simulink model "Wheelspeed_Logik_compatible"  (R2022b)
settings: Solver=FixedStepAuto  StartTime=0.0  StopTime=10.0  FixedStep=0.0001  RelTol=1e-3
libraries: simulink x2
settings Model: Creator=finneinhoff  LastModifiedBy=finneinhoff
settings OptimizationCC: ReuseModelBlockBuffer=on
settings RTWCC: GPUComputeCapability=5.0
settings ConfigComp: CovBoundaryAbsTol=1.0e-5

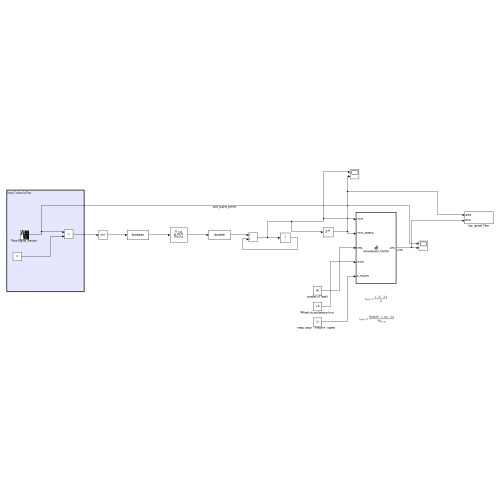
[thumbnail: Simulink's stored preview of the top-level diagram]
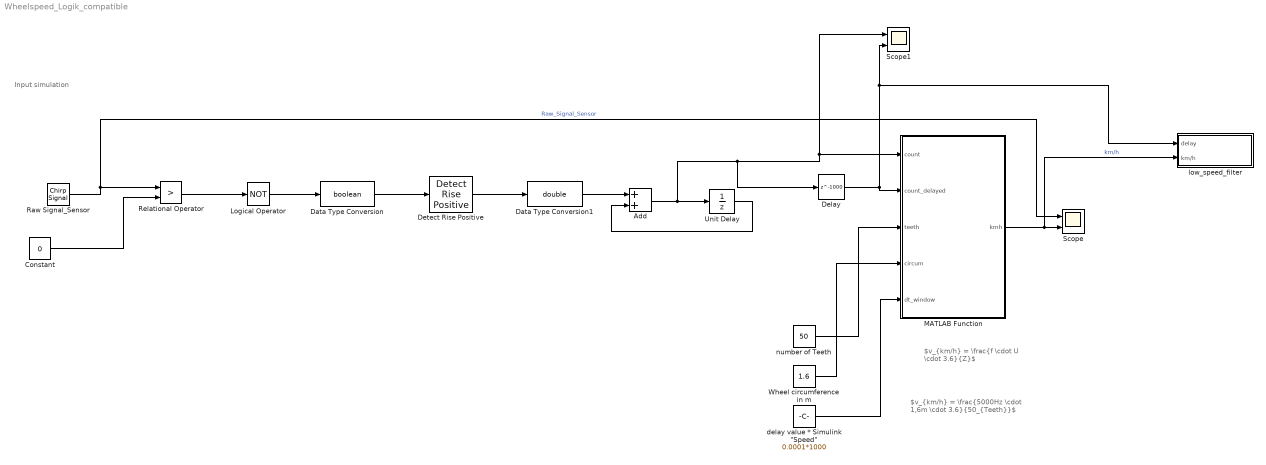
== system Wheelspeed_Logik_compatible ==
  note: Input simulation
  note: $v_{km/h} = \frac{5000Hz \cdot 1,6m \cdot 3.6}{50_{Teeth}}$
  note: $v_{km/h} = \frac{f \cdot U \cdot 3.6}{Z}$
  Add : Sum  OutDataTypeStr=double
  Constant : Constant  Value=0
  Data Type Conversion : DataTypeConversion  OutDataTypeStr=boolean  SaturateOnIntegerOverflow=off  RndMeth=Floor
  Data Type Conversion1 : DataTypeConversion  OutDataTypeStr=double  SaturateOnIntegerOverflow=off  RndMeth=Floor
  Delay : Delay  DelayLength=1000
  Detect Rise Positive : simulink/Logic and Bit Operations/Detect Rise Positive  vinit=0  OutDataTypeStr=boolean
  Logical Operator : Logic  Operator=NOT  AllPortsSameDT=off  OutDataTypeStr=boolean
  MATLAB Function : MATLAB Function  TreatAsAtomicUnit=on
  Raw Signal_Sensor : simulink/Sources/Chirp Signal  f1=10  T=10  f2=5000
  Relational Operator : RelationalOperator  Operator=>  OutDataTypeStr=boolean  RndMeth=Simplest  InputSameDT=off
  Scope : Scope  NumInputPorts=2
  Scope1 : Scope  NumInputPorts=2
  Unit Delay : UnitDelay  SampleTime=-1  HasFrameUpgradeWarning=on
  Wheel circumference in m : Constant  Value=1.6
  "delay value * Simulink \"Speed\" " : Constant  Value=0.0001*1000
  low_speed_filter : Subsystem
  number of Teeth : Constant  Value=50
  wires:
  Logical Operator/1 -> Data Type Conversion/1
  Detect Rise Positive/1 -> Data Type Conversion1/1
  Add/1 -> Scope1/1, MATLAB Function/1(count), Delay/1, Unit Delay/1
  Unit Delay/1 -> Add/2
  number of Teeth/1 -> MATLAB Function/3(teeth)
  Wheel circumference in m/1 -> MATLAB Function/4(circum)
  "delay value * Simulink \"Speed\" "/1 -> MATLAB Function/5(dt_window)
  Raw Signal_Sensor/1 -> Relational Operator/1, Scope/1  "Raw_Signal_Sensor"
  Relational Operator/1 -> Logical Operator/1
  MATLAB Function/1(kmh) -> low_speed_filter/2(km/h), Scope/2  "km/h"
  Constant/1 -> Relational Operator/2
  Data Type Conversion1/1 -> Add/1
  Delay/1 -> MATLAB Function/2(count_delayed), low_speed_filter/1(delay), Scope1/2
  Data Type Conversion/1 -> Detect Rise Positive/1

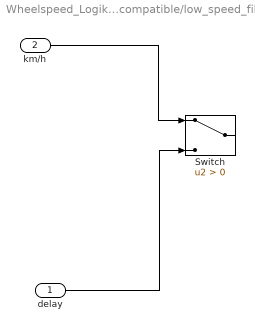
== system Wheelspeed_Logik_compatible/low_speed_filter ==
  delay : Inport
  km/h : Inport  Port=2
  Switch : Switch  Criteria=u2 > Threshold  SaturateOnIntegerOverflow=off  InputSameDT=off
  wires:
  delay/1 -> Switch/3
  km/h/1 -> Switch/1

== matlab function Wheelspeed_Logik_compatible/MATLAB Function ==
  data: count input; kmh output; count_delayed input; teeth input; circum input; dt_window input
function kmh = wheelspeed_fs2026(count, count_delayed, teeth, circum, dt_window)
    persistent last_kmh;
    if isempty(last_kmh)
        last_kmh = 0;
    end

    c1 = double(count);
    c0 = double(count_delayed);
    
    % Wenn der Zähler sich nicht bewegt hat, halten wir den alten Wert
    % oder berechnen den neuen Durchschnitt
    delta = c1 - c0;
    
    if double(dt_window) > 0
        new_kmh = (delta / double(dt_window) / double(teeth)) * double(circum) * 3.6;
        kmh = new_kmh;
        last_kmh = new_kmh;
    else
        kmh = last_kmh;
    end
end
